simulink model "Lab1_419_simul4"  (R2023b)
settings: Solver=VariableStepAuto  StartTime=0.0  StopTime=30  RelTol=1e-3
settings Model: Creator=Aiden  LastModifiedBy=julia

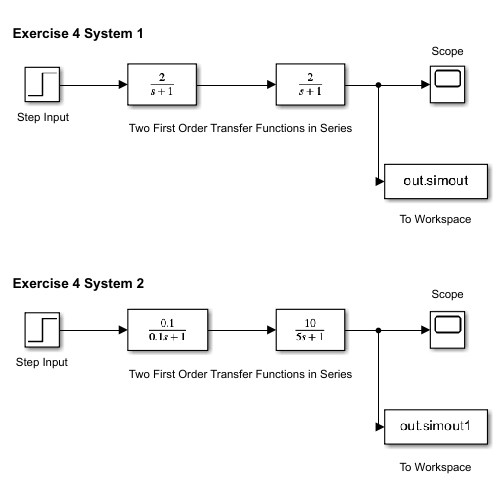
[thumbnail: Simulink's stored preview of the top-level diagram]
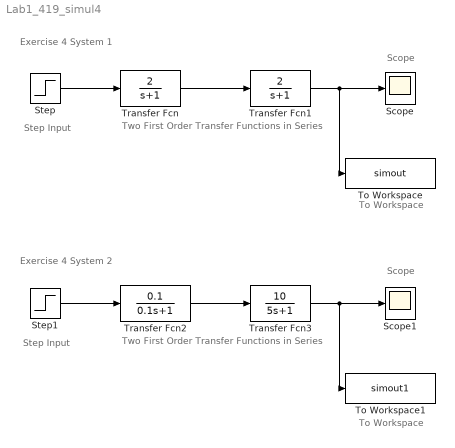
== system Lab1_419_simul4 ==
  note: Step Input
  note: Two First Order Transfer Functions in Series
  note: Scope
  note: To Workspace
  note: Exercise 4 System 1
  note: Exercise 4 System 2
  note: To Workspace
  note: Scope
  note: Two First Order Transfer Functions in Series
  note: Step Input
  Scope : Scope
  Scope1 : Scope
  Step : Step  SampleTime=0
  Step1 : Step  SampleTime=0
  To Workspace : ToWorkspace  VariableName=simout  SampleTime=-1
  To Workspace1 : ToWorkspace  VariableName=simout1  SampleTime=-1
  Transfer Fcn : TransferFcn  Numerator=[2]  Denominator=[1 1]
  Transfer Fcn1 : TransferFcn  Numerator=[2]  Denominator=[1 1]
  Transfer Fcn2 : TransferFcn  Numerator=[0.1]  Denominator=[0.1 1]
  Transfer Fcn3 : TransferFcn  Numerator=[10]  Denominator=[5 1]
  wires:
  Step/1 -> Transfer Fcn/1
  Transfer Fcn/1 -> Transfer Fcn1/1
  Transfer Fcn1/1 -> To Workspace/1, Scope/1
  Transfer Fcn3/1 -> Scope1/1, To Workspace1/1
  Step1/1 -> Transfer Fcn2/1
  Transfer Fcn2/1 -> Transfer Fcn3/1
